simulink library "library"  (Simulink 9.1)
settings: Solver=ode45  StartTime=0.0  StopTime=10.0  RelTol=1e-3  EnableMultiTasking=on
undefined symbols (not defined in the file or in its folder): contr, curvature, k, l, pin, sysCtrl
libraries: $bdroot x15, cstblocks x1
(part 2 of 2)

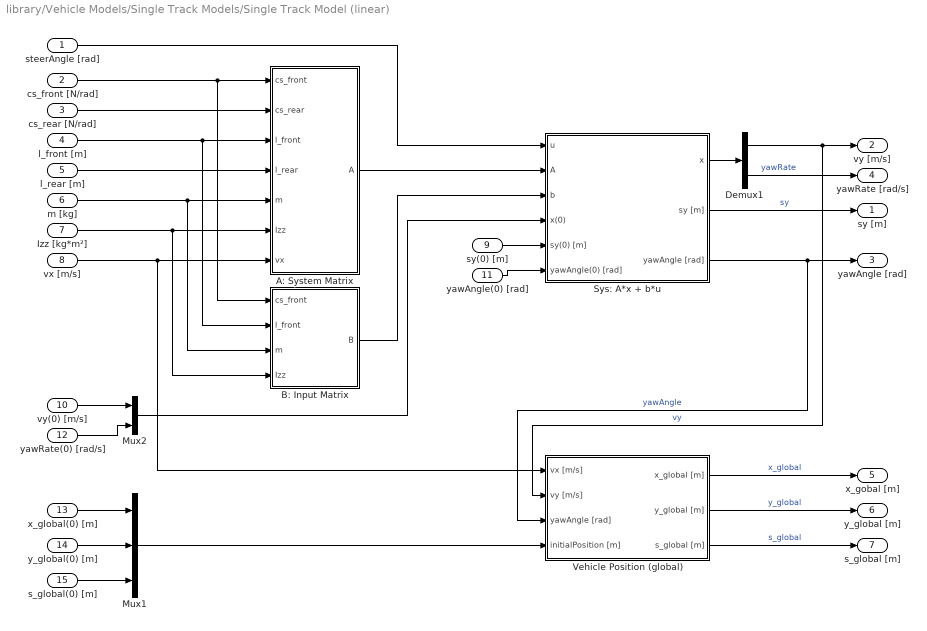
== system library/Vehicle Models/Single Track Models/Single Track Model (linear) ==
  steerAngle [rad] : Inport  OutDataTypeStr=double  PortDimensions=1
  cs_front [N/rad] : Inport  Port=2  OutDataTypeStr=double  PortDimensions=1
  cs_rear [N/rad] : Inport  Port=3  OutDataTypeStr=double  PortDimensions=1
  l_front [m] : Inport  Port=4  OutMin=0  OutDataTypeStr=double  PortDimensions=1
  l_rear [m] : Inport  Port=5  OutMin=0  OutDataTypeStr=double  PortDimensions=1
  m [kg] : Inport  Port=6  OutMin=0  OutDataTypeStr=double  PortDimensions=1
  Izz [kg*m²] : Inport  Port=7  OutMin=0  OutDataTypeStr=double  PortDimensions=1
  vx [m/s] : Inport  Port=8  OutDataTypeStr=double  PortDimensions=1
  sy(0) [m] : Inport  Port=9  OutDataTypeStr=double  PortDimensions=1
  vy(0) [m/s] : Inport  Port=10  OutDataTypeStr=double  PortDimensions=1
  yawAngle(0) [rad] : Inport  Port=11  OutDataTypeStr=double  PortDimensions=1
  yawRate(0) [rad/s] : Inport  Port=12  OutDataTypeStr=double  PortDimensions=1
  x_global(0) [m] : Inport  Port=13  OutDataTypeStr=double  PortDimensions=1
  y_global(0) [m] : Inport  Port=14  OutDataTypeStr=double  PortDimensions=1
  s_global(0) [m] : Inport  Port=15  OutDataTypeStr=double  PortDimensions=1
  A: System Matrix : Subsystem
  B: Input Matrix : Subsystem
  Demux1 : Demux  Outputs=2
  Mux1 : Mux  Inputs=3
  Mux2 : Mux  Inputs=2
  Sys: A*x + b*u : Subsystem
  Vehicle Position (global) : Subsystem
  sy [m] : Outport  OutDataTypeStr=double  PortDimensions=1
  vy [m/s] : Outport  Port=2  OutDataTypeStr=double  PortDimensions=1
  yawAngle [rad] : Outport  Port=3  OutDataTypeStr=double  PortDimensions=1
  yawRate [rad/s] : Outport  Port=4  OutDataTypeStr=double  PortDimensions=1
  x_gobal [m] : Outport  Port=5  OutDataTypeStr=double  PortDimensions=1
  y_global [m] : Outport  Port=6  OutDataTypeStr=double  PortDimensions=1
  s_global [m] : Outport  Port=7  OutDataTypeStr=double  PortDimensions=1
  wires:
  steerAngle [rad]/1 -> Sys: A*x + b*u/1(u)
  cs_front [N/rad]/1 -> A: System Matrix/1(cs_front), B: Input Matrix/1(cs_front)
  cs_rear [N/rad]/1 -> A: System Matrix/2(cs_rear)
  l_front [m]/1 -> A: System Matrix/3(l_front), B: Input Matrix/2(l_front)
  l_rear [m]/1 -> A: System Matrix/4(l_rear)
  m [kg]/1 -> A: System Matrix/5(m), B: Input Matrix/3(m)
  Izz [kg*m²]/1 -> A: System Matrix/6(Izz), B: Input Matrix/4(Izz)
  vx [m/s]/1 -> A: System Matrix/7(vx), Vehicle Position (global)/1(vx [m/s])
  Sys: A*x + b*u/2(sy [m]) -> sy [m]/1  "sy"
  Sys: A*x + b*u/3(yawAngle [rad]) -> yawAngle [rad]/1, Vehicle Position (global)/3(yawAngle [rad])  "yawAngle"
  Demux1/2 -> yawRate [rad/s]/1  "yawRate"
  Vehicle Position (global)/1(x_global [m]) -> x_gobal [m]/1  "x_global"
  Vehicle Position (global)/2(y_global [m]) -> y_global [m]/1  "y_global"
  Vehicle Position (global)/3(s_global [m]) -> s_global [m]/1  "s_global"
  vy(0) [m/s]/1 -> Mux2/1
  yawRate(0) [rad/s]/1 -> Mux2/2
  x_global(0) [m]/1 -> Mux1/1
  y_global(0) [m]/1 -> Mux1/2
  s_global(0) [m]/1 -> Mux1/3
  Mux1/1 -> Vehicle Position (global)/4(initialPosition [m])
  A: System Matrix/1(A) -> Sys: A*x + b*u/2(A)
  B: Input Matrix/1(B) -> Sys: A*x + b*u/3(b)
  Mux2/1 -> Sys: A*x + b*u/4(x(0))
  sy(0) [m]/1 -> Sys: A*x + b*u/5(sy(0) [m])
  yawAngle(0) [rad]/1 -> Sys: A*x + b*u/6(yawAngle(0) [rad])
  Sys: A*x + b*u/1(x) -> Demux1/1
  Demux1/1 -> vy [m/s]/1, Vehicle Position (global)/2(vy [m/s])  "vy"

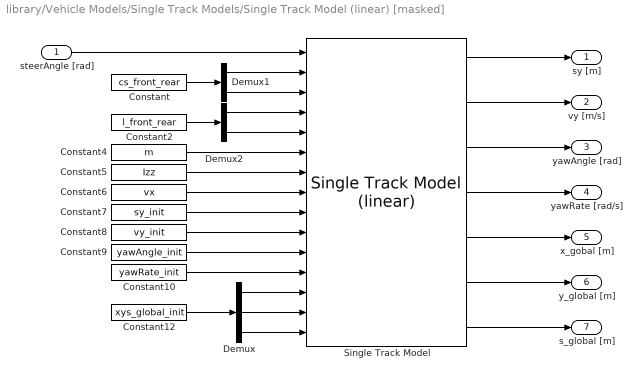
== system library/Vehicle Models/Single Track Models/Single Track Model (linear) [masked] ==
  steerAngle [rad] : Inport
  Constant : Constant  Value=cs_front_rear
  Constant10 : Constant  Value=yawRate_init
  Constant12 : Constant  Value=xys_global_init
  Constant2 : Constant  Value=l_front_rear
  Constant4 : Constant  Value=m
  Constant5 : Constant  Value=Izz
  Constant6 : Constant  Value=vx
  Constant7 : Constant  Value=sy_init
  Constant8 : Constant  Value=vy_init
  Constant9 : Constant  Value=yawAngle_init
  Demux : Demux  Outputs=3
  Demux1 : Demux  Outputs=2
  Demux2 : Demux  Outputs=2
  Single Track Model : $bdroot/Vehicle Models/Single Track Models/Single Track Model (linear)
  sy [m] : Outport
  vy [m/s] : Outport  Port=2
  yawAngle [rad] : Outport  Port=3
  yawRate [rad/s] : Outport  Port=4
  x_gobal [m] : Outport  Port=5
  y_global [m] : Outport  Port=6
  s_global [m] : Outport  Port=7
  wires:
  steerAngle [rad]/1 -> Single Track Model/1
  Constant4/1 -> Single Track Model/6
  Constant5/1 -> Single Track Model/7
  Constant6/1 -> Single Track Model/8
  Single Track Model/1 -> sy [m]/1
  Single Track Model/2 -> vy [m/s]/1
  Single Track Model/3 -> yawAngle [rad]/1
  Single Track Model/4 -> yawRate [rad/s]/1
  Single Track Model/5 -> x_gobal [m]/1
  Single Track Model/6 -> y_global [m]/1
  Single Track Model/7 -> s_global [m]/1
  Constant7/1 -> Single Track Model/9
  Constant8/1 -> Single Track Model/10
  Constant9/1 -> Single Track Model/11
  Constant10/1 -> Single Track Model/12
  Constant12/1 -> Demux/1
  Demux/1 -> Single Track Model/13
  Demux/2 -> Single Track Model/14
  Demux/3 -> Single Track Model/15
  Demux1/1 -> Single Track Model/2
  Demux1/2 -> Single Track Model/3
  Constant/1 -> Demux1/1
  Demux2/1 -> Single Track Model/4
  Demux2/2 -> Single Track Model/5
  Constant2/1 -> Demux2/1

== system library/Vehicle Models/Single Track Models/Single Track Model (linear)/A: System Matrix ==
  cs_front : Inport
  cs_rear : Inport  Port=2
  l_front : Inport  Port=3
  l_rear : Inport  Port=4
  m : Inport  Port=5
  Izz : Inport  Port=6
  vx : Inport  Port=7
  Coeffiecient a11 : Subsystem
  Coeffiecient a12 : Subsystem
  Coeffiecient a21 : Subsystem
  Coeffiecient a22 : Subsystem
  Mux : Mux  Inputs=2
  Mux1 : Mux  Inputs=2
  Vector Concatenate : Concatenate  Mode=Multidimensional array  ConcatenateDimension=2
  A : Outport
  wires:
  cs_front/1 -> Coeffiecient a11/1(csv), Coeffiecient a12/1(csv), Coeffiecient a21/1(csv), Coeffiecient a22/1(csv)
  cs_rear/1 -> Coeffiecient a11/2(csh), Coeffiecient a12/2(csh), Coeffiecient a21/2(csh), Coeffiecient a22/2(csh)
  m/1 -> Coeffiecient a11/3(m), Coeffiecient a12/5(m)
  vx/1 -> Coeffiecient a11/4(vx), Coeffiecient a12/6(vx), Coeffiecient a21/6(vx), Coeffiecient a22/6(vx)
  l_front/1 -> Coeffiecient a12/3(lv), Coeffiecient a21/3(lv), Coeffiecient a22/3(lv)
  l_rear/1 -> Coeffiecient a12/4(lh), Coeffiecient a22/4(lh), Coeffiecient a21/4(lh)
  Izz/1 -> Coeffiecient a21/5(Izz), Coeffiecient a22/5(Izz)
  Coeffiecient a11/1(a11) -> Mux/1
  Coeffiecient a22/1(a22) -> Mux1/2
  Mux/1 -> Vector Concatenate/1
  Mux1/1 -> Vector Concatenate/2
  Vector Concatenate/1 -> A/1  "A"
  Coeffiecient a12/1(a12) -> Mux1/1
  Coeffiecient a21/1(a21) -> Mux/2

== system library/Vehicle Models/Single Track Models/Single Track Model (linear)/B: Input Matrix ==
  cs_front : Inport
  l_front : Inport  Port=2
  m : Inport  Port=3
  Izz : Inport  Port=4
  Divide : Product  Inputs=*/
  Divide1 : Product  Inputs=**/
  Mux : Mux  Inputs=2
  B : Outport
  wires:
  cs_front/1 -> Divide/1, Divide1/1
  m/1 -> Divide/2
  Izz/1 -> Divide1/3
  l_front/1 -> Divide1/2
  Divide/1 -> Mux/1
  Divide1/1 -> Mux/2
  Mux/1 -> B/1

== system library/Vehicle Models/Single Track Models/Single Track Model (linear)/Sys: A*x + b*u ==
  u : Inport
  A : Inport  Port=2
  b : Inport  Port=3
  x(0) : Inport  Port=4
  sy(0) [m] : Inport  Port=5  OutDataTypeStr=double  PortDimensions=1
  yawAngle(0) [rad] : Inport  Port=6  OutDataTypeStr=double  PortDimensions=1
  A*x : Product  Multiplication=Matrix(*)  RndMeth=Zero
  Demux1 : Demux  Outputs=2
  Integrator1 : Integrator  InitialConditionSource=external
  Integrator2 : Integrator  InitialConditionSource=external
  Mux2 : Mux  Inputs=2
  Sum : Sum  Inputs=++|
  b*u : Product  Multiplication=Matrix(*)  RndMeth=Zero
  x : Outport  OutDataTypeStr=double  PortDimensions=2
  sy [m] : Outport  Port=2  OutDataTypeStr=double  PortDimensions=1
  yawAngle [rad] : Outport  Port=3  OutDataTypeStr=double  PortDimensions=1
  wires:
  Sum/1 -> Integrator1/1
  Integrator1/1 -> A*x/2, Integrator2/1, x/1
  A/1 -> A*x/1
  x(0)/1 -> Integrator1/2
  b/1 -> b*u/1
  u/1 -> b*u/2
  A*x/1 -> Sum/2
  b*u/1 -> Sum/1
  sy(0) [m]/1 -> Mux2/1
  yawAngle(0) [rad]/1 -> Mux2/2
  Mux2/1 -> Integrator2/2
  Integrator2/1 -> Demux1/1
  Demux1/1 -> sy [m]/1
  Demux1/2 -> yawAngle [rad]/1

== system library/Vehicle Models/Single Track Models/Single Track Model (linear)/Vehicle Position (global) ==
  vx [m/s] : Inport
  vy [m/s] : Inport  Port=2
  yawAngle [rad] : Inport  Port=3
  initialPosition [m] : Inport  Port=4
  Demux : Demux  Outputs=3
  Fcn1 : Fcn  Expr=u(1)*cos(u(3)) - u(2)*sin(u(3))
  Fcn2 : Fcn  Expr=u(1)*sin(u(3)) + u(2)*cos(u(3))
  Fcn3 : Fcn  Expr=sqrt( u(1)^2 + u(2)^2 )
  Integrator1 : Integrator  InitialConditionSource=external
  Integrator2 : Integrator  InitialConditionSource=external
  Integrator3 : Integrator  InitialConditionSource=external
  Mux : Mux  Inputs=3
  x_global [m] : Outport
  y_global [m] : Outport  Port=2
  s_global [m] : Outport  Port=3
  wires:
  Integrator2/1 -> y_global [m]/1
  yawAngle [rad]/1 -> Mux/3
  vy [m/s]/1 -> Mux/2
  vx [m/s]/1 -> Mux/1
  Integrator1/1 -> x_global [m]/1
  Fcn2/1 -> Integrator2/1
  Fcn1/1 -> Integrator1/1
  Fcn3/1 -> Integrator3/1
  Integrator3/1 -> s_global [m]/1
  Mux/1 -> Fcn2/1, Fcn1/1, Fcn3/1
  initialPosition [m]/1 -> Demux/1
  Demux/1 -> Integrator1/2
  Demux/2 -> Integrator2/2
  Demux/3 -> Integrator3/2

== system library/Vehicle Models/Single Track Models/Single Track Model (linear)/A: System Matrix/Coeffiecient a11 ==
  csv : Inport
  csh : Inport  Port=2
  m : Inport  Port=3
  vx : Inport  Port=4
  Add : Sum
  Divide2 : Product  Inputs=*//
  Gain : Gain  Gain=-1
  a11 : Outport
  wires:
  Add/1 -> Divide2/1
  csv/1 -> Add/1
  csh/1 -> Add/2
  m/1 -> Divide2/2
  Divide2/1 -> Gain/1
  vx/1 -> Divide2/3
  Gain/1 -> a11/1

== system library/Vehicle Models/Single Track Models/Single Track Model (linear)/A: System Matrix/Coeffiecient a12 ==
  csv : Inport
  csh : Inport  Port=2
  lv : Inport  Port=3
  lh : Inport  Port=4
  m : Inport  Port=5
  vx : Inport  Port=6
  Add1 : Sum  Inputs=+-
  Add2 : Sum  Inputs=-+
  Divide : Product  Inputs=*/
  Product : Product  RndMeth=Zero
  Product1 : Product  RndMeth=Zero
  Product2 : Product  RndMeth=Zero
  a12 : Outport
  wires:
  csv/1 -> Product/1
  Add1/1 -> a12/1
  lv/1 -> Product/2
  csh/1 -> Product1/1
  lh/1 -> Product1/2
  Product/1 -> Add2/1
  Product1/1 -> Add2/2
  Add2/1 -> Divide/1
  m/1 -> Product2/1
  vx/1 -> Product2/2, Add1/2
  Product2/1 -> Divide/2
  Divide/1 -> Add1/1

== system library/Vehicle Models/Single Track Models/Single Track Model (linear)/A: System Matrix/Coeffiecient a21 ==
  csv : Inport
  csh : Inport  Port=2
  lv : Inport  Port=3
  lh : Inport  Port=4
  Izz : Inport  Port=5
  vx : Inport  Port=6
  Add2 : Sum  Inputs=-+
  Divide : Product  Inputs=*/
  Product : Product  RndMeth=Zero
  Product1 : Product  RndMeth=Zero
  Product2 : Product  RndMeth=Zero
  a21 : Outport
  wires:
  Product2/1 -> Divide/2
  vx/1 -> Product2/2
  Izz/1 -> Product2/1
  Add2/1 -> Divide/1
  Product1/1 -> Add2/2
  Product/1 -> Add2/1
  lh/1 -> Product1/2
  csh/1 -> Product1/1
  lv/1 -> Product/2
  Divide/1 -> a21/1
  csv/1 -> Product/1

== system library/Vehicle Models/Single Track Models/Single Track Model (linear)/A: System Matrix/Coeffiecient a22 ==
  csv : Inport
  csh : Inport  Port=2
  lv : Inport  Port=3
  lh : Inport  Port=4
  Izz : Inport  Port=5
  vx : Inport  Port=6
  Add2 : Sum
  Divide : Product  Inputs=*/
  Gain : Gain  Gain=-1
  Math Function : Math  Operator=square  SaturateOnIntegerOverflow=on
  Math Function1 : Math  Operator=square  SaturateOnIntegerOverflow=on
  Product : Product  RndMeth=Zero
  Product1 : Product  RndMeth=Zero
  Product2 : Product  RndMeth=Zero
  a22 : Outport
  wires:
  csv/1 -> Product/1
  Divide/1 -> Gain/1
  lv/1 -> Math Function/1
  csh/1 -> Product1/1
  lh/1 -> Math Function1/1
  Product/1 -> Add2/1
  Product1/1 -> Add2/2
  Add2/1 -> Divide/1
  Izz/1 -> Product2/1
  vx/1 -> Product2/2
  Product2/1 -> Divide/2
  Math Function/1 -> Product/2
  Math Function1/1 -> Product1/2
  Gain/1 -> a22/1

== matlab function Lane Tracking/Lane Tracking Sensor/MATLAB Function ==
  data: LAD input double; isValid_LAD input double; lateralOff_LAD input double; angularDev_LAD input double; roadCurvat_LAD input double; poly_lateralOff_LAD output double; poly_angularDev_LAD output double; poly_roadCurvat_LAD output double; poly_domain_LAD output double
function [...
 poly_lateralOff_LAD,...
 poly_angularDev_LAD,...
 poly_roadCurvat_LAD,...
 poly_domain_LAD] = polyFitLaneSensor(...
 LAD,...
 isValid_LAD,...
 lateralOff_LAD,...
 angularDev_LAD,...
 roadCurvat_LAD)
%#codegen


%%% number of valid measurements specify maximum degree of polynomial
np_max = sum(isValid_LAD) - 1;

if any(~isValid_LAD)
	1;
end%if

%%% init outputs
% choose polynomial degree/fixed output length
np = 3;
poly_lateralOff_LAD	= zeros(1,np+1);
poly_angularDev_LAD	= zeros(1,np+1);
poly_roadCurvat_LAD	= zeros(1,np+1);

%%% fit polynomial coefficients
n = min(np,np_max);
LAD_valid = LAD(isValid_LAD);
poly_latOff	= polyfit(LAD_valid,lateralOff_LAD(isValid_LAD),n);
poly_angDev	= polyfit(LAD_valid,angularDev_LAD(isValid_LAD),n);
poly_rdCurv	= polyfit(LAD_valid,roadCurvat_LAD(isValid_LAD),n);

%%% add coefficients to output
poly_lateralOff_LAD(np-n+1:np+1) = poly_latOff;
poly_angularDev_LAD(np-n+1:np+1) = poly_angDev;
poly_roadCurvat_LAD(np-n+1:np+1) = poly_rdCurv;

poly_domain_LAD = [min(LAD_valid);max(LAD_valid)];

end%fcn
